simulink library "tqd"  (R2021b)
settings: Solver=VariableStepAuto  StartTime=0.0  StopTime=10.0  RelTol=1e-3
undefined symbols (not defined in the file or in its folder): ATQD_APSDecReq_X_kph, ATQD_APSDecReq_Y_mps2, ATQD_APSDecReqCMD_X_kph, ATQD_APSDecReqTs_X_pct, ATQD_APSDecTimeGain_X_Deg, ATQD_APSDecTimeGain_Y_s, ATQD_APSReqLowSpd_X_Deg, ATQD_AutoHoldReleaseBPS_X_Deg, ATQD_AWDLoadTrqnsGain_X_kg, ATQD_AWDLoadTrqnsGain_Y_pct, ATQD_BOSEnBPSPosn_X_kph, ATQD_BOSMap_X_rpm, ATQD_BOSMap_Y_pct, ATQD_CreepBaseTqD_X_kph, ATQD_CreepBaseTqD_Y_Deg, ATQD_CreepBaseTqR_X_kph, ATQD_CreepBaseTqR_Y_Deg, ATQD_CreepBPSDisPosn_X_Deg, ATQD_CreepBPSDisPosnR_X_Deg, ATQD_CreepBPSEnPosn_X_Deg, ATQD_CreepBPSEnPosnR_X_Deg, ATQD_CreepDeltaTq_X_kph, ATQD_CreepIterm_X_kph, ATQD_CreepIterm_Y_kph, ATQD_CreepItermMaxLimit_X_pct, ATQD_CreepPreloadTime_X_kph, ATQD_CreepPreloadTq_X_kph, ATQD_CreepPreloadTq_Y_s, ATQD_CreepProtTq_X_Deg, ATQD_CreepPterm_X_kph, ATQD_ECOTqMapD_X_rpm, ATQD_ECOTqMapD_Y_pct, ATQD_EOPDTqMapDCon_X_rpm, ATQD_EOPDTqMapDCon_Y_Deg, ATQD_EstInitVehWeight_X_c, ATQD_LHMRollGenMapD_X_rpm, ATQD_LHMRollGenMapD_Y_rpm, ATQD_LHMTqMapD_X_rpm, ATQD_LHMTqMapD_Y_pct, ATQD_NL1TqMapD_X_rpm, ATQD_NL1TqMapD_Y_pct, ATQD_NOPDTqMapDCon_X_rpm, ATQD_NOPDTqMapDCon_Y_Deg, ATQD_NRMRrEDUSpRat_X_rpm, ATQD_NRMRrEDUSpRat_Y_Nm, ATQD_OPDHoldDownRelDelay_X_Deg, ATQD_OPDHoldEnSpd_X_Deg, ATQD_OPDHoldRelDetTime_X_Deg, ATQD_OPDHoldReleaseTq_X_Deg, ATQD_OrigPedTqLowLim_X_Deg, ATQD_OrigPedTqLowLim_Y_pct, ATQD_PedalMapClimbUpLim_X_rpm, ATQD_PedalMapClimbUpLim_Y_Deg, ATQD_PreLoadTq_X_s, ATQD_RollGenMapEL1_X_rpm, ATQD_RollGenMapEL1_Y_rpm, ATQD_SL1TqMapD_X_rpm, ATQD_SL1TqMapD_Y_pct, ATQD_SlideRegenTqGain_X_Gps, ATQD_SlideRegenTqGain_Y_pct ... (+378)
libraries: hcu_lib x59, simulink x49
(part 3 of 12)

== system tqd/TQD/TorqueDemand/ShiftModule ==
  task_time_s : Inport
  VINP_ShifterHandleCmd_enum : Inport  Port=2
  VINP_VehSpeed_kph : Inport  Port=3
  VTQD_BrkSwSta_flg : Inport  Port=4
  VPMM_PowerSta_enum : Inport  Port=5
  VINP_PBWMotorPos_enum : Inport  Port=6
  VTQD_TMRotateDirction_enum : Inport  Port=7
  VTQD_EPBCarWashMode_flg : Inport  Port=8
  VINP_DrDoorSW_flg : Inport  Port=9
  VVMC_APSShiftPosnReq_enum : Inport  Port=10
  VVMC_APSActive_flg : Inport  Port=11
  VINP_DriverSeatBeltCmd_flg : Inport  Port=12
  VINP_SeatSW_flg : Inport  Port=13
  VINP_ChrgPlugSta_enum : Inport  Port=14
  VINP_SCPSystemMode_enum : Inport  Port=15
  VTQD_AfterAvailableTqDemFr_Nm : Inport  Port=16
  VTQD_AfterAvailableTqDemRr_Nm : Inport  Port=17
  VTQR_NoABSFEDUWhlTqReq_Nm : Inport  Port=18
  VTQR_NoABSREDUWhlTqReq_Nm : Inport  Port=19
  VINP_DOASta_flg : Inport  Port=20
  VTQD_IVIPwrLock_flg : Inport  Port=21
  VTQD_OPDHoldAllowPark_flg : Inport  Port=22
  Constant : Constant  Value=KTQD_VehSpd2P_kph
  Constant1 : Constant  Value=KTQD_PBWTimeout_s
  Constant2 : Constant  Value=KTQD_VehSpdRev_kph
  Constant3 : Constant  Value=KTQD_ShiftInitialTime_s
  Constant4 : Constant  Value=KTQD_RelockWaitTime_s
  Constant5 : Constant  Value=KTQD_ReunlockWaitTime_s
  Constant6 : Constant  Value=ENUM_GEARACTUALPOSN_P
  Constant7 : Constant  Value=ENUM_GEARACTUALPOSN_P
  Data Type Conversion1 : DataTypeConversion
  Data Type Conversion2 : DataTypeConversion
  Data Type Conversion3 : DataTypeConversion  OutDataTypeStr=uint8
  Data Type Conversion4 : DataTypeConversion  OutDataTypeStr=boolean
  Determine_Actual_Gear_Position : Stateflow chart  TreatAsAtomicUnit=on
  Equal : RelationalOperator  Operator===  OutDataTypeStr=boolean  RndMeth=Simplest
  Equal1 : RelationalOperator  Operator=~=  OutDataTypeStr=boolean  RndMeth=Simplest
  GearShiftPosn : Subsystem  Description=GearPosition
  P_Button_State_Judge : Subsystem
  SR_Latch : hcu_lib/Basic_Blocks/SR_Latch
  SR_Latch1 : Subsystem  mask(SR_Latch){}
      mask help: SR latch function.
  Terminator : Terminator
  VTQD_GearActualPosn_enum : Outport
  VTQD_ParkRequest_flg : Outport  Port=2
  VTQD_PBWLockTO_flg : Outport  Port=3
  VTQD_PBWUnlockTO_flg : Outport  Port=4
  VTQD_PButtonSta_enum : Outport  Port=5
  VTQD_DriveProtRemove_flg : Outport  Port=6
  VTQD_DriveProtEn_flg : Outport  Port=7
  wires:
  VPMM_PowerSta_enum/1 -> [VPMM_PowerSta_enum]
  task_time_s/1 -> [task_time_s]
  VINP_VehSpeed_kph/1 -> [VINP_VehSpeed_kph]
  VTQD_BrkSwSta_flg/1 -> [VTQD_BrkSwSta_flg]
  VTQD_TMRotateDirction_enum/1 -> [VTQD_TMRotateDirction_enum]
  VINP_PBWMotorPos_enum/1 -> [VINP_PBWMotorPos_enum]
  P_Button_State_Judge/1(VTQD_PButtonSta_enum) -> VTQD_PButtonSta_enum/1
  VINP_ShifterHandleCmd_enum/1 -> [VINP_ShifterHandleCmd_enum]
  [VINP_ShifterHandleCmd_enum] -> P_Button_State_Judge/1(VINP_ShifterHandleCmd_enum)
  VINP_SCPSystemMode_enum/1 -> Terminator/1
  VINP_ChrgPlugSta_enum/1 -> [VINP_ChrgPlugSta_enum]
  VINP_SeatSW_flg/1 -> [VINP_SeatSW_flg]
  VINP_DriverSeatBeltCmd_flg/1 -> [VINP_DriverSeatBeltCmd_flg]
  VVMC_APSActive_flg/1 -> [VVMC_APSActive_flg]
  VVMC_APSShiftPosnReq_enum/1 -> [VVMC_APSShiftPosnReq_enum]
  VINP_DrDoorSW_flg/1 -> [VINP_DrDoorSW_flg]
  VTQD_EPBCarWashMode_flg/1 -> [VTQD_EPBCarWashMode_flg]
  [VTQD_EPBCarWashMode_flg] -> GearShiftPosn/8(VTQD_EPBCarWashMode_flg)
  [VINP_VehSpeed_kph] -> GearShiftPosn/9(VINP_VehSpeed_kph)
  [VINP_ChrgPlugSta_enum] -> GearShiftPosn/10(VINP_ChrgPlugSta_enum)
  GearShiftPosn/3(VTQD_PwrStaAllowDR_flg) -> [VTQD_PwrStaAllowDR_flg]
  [VVMC_APSShiftPosnReq_enum] -> GearShiftPosn/4(VVMC_APSShiftPosnReq_enum)
  [VINP_DrDoorSW_flg] -> GearShiftPosn/3(VINP_DrDoorSW_flg)
  [VINP_ShifterHandleCmd_enum] -> GearShiftPosn/1(VINP_ShifterHandleCmd_enum)
  [VVMC_APSActive_flg] -> GearShiftPosn/5(VVMC_APSActive_flg)
  [VINP_DriverSeatBeltCmd_flg] -> GearShiftPosn/6(VINP_DriverSeatBeltCmd_flg)
  GearShiftPosn/1(VTQD_GearShiftCMD_enum) -> [VTQD_GearShiftCMD_enum]
  [VINP_SeatSW_flg] -> GearShiftPosn/7(VINP_SeatSW_flg)
  [VPMM_PowerSta_enum] -> GearShiftPosn/2(VPMM_PowerSta_enum)
  GearShiftPosn/2(VTQD_PwrStaAllowPN_flg) -> [VTQD_PwrStaAllowPN_flg]
  Data Type Conversion4/1 -> VTQD_ParkRequest_flg/1  "VTQD_ParkRequest_flg"
  Constant6/1 -> Equal/2
  Data Type Conversion1/1 -> SR_Latch/1
  [VTQD_GearActualPosn_enum] -> Equal1/1
  [VTQD_GearActualPosn_enum] -> Equal/1
  Data Type Conversion2/1 -> SR_Latch1/1(set)
  Determine_Actual_Gear_Position/4(VTQD_ParkRequest_flg) -> Data Type Conversion4/1
  Constant7/1 -> Equal1/2
  Data Type Conversion3/1 -> [VTQD_GearActualPosn_enum], VTQD_GearActualPosn_enum/1  "VTQD_GearActualPosn_enum"
  Determine_Actual_Gear_Position/3(VTQD_PBWUnlockTO_flg) -> Data Type Conversion2/1
  SR_Latch1/1(latched) -> VTQD_PBWUnlockTO_flg/1  "VTQD_PBWUnlockTO_flg"
  Equal1/1 -> SR_Latch1/2(reset)
  Equal/1 -> SR_Latch/2
  Determine_Actual_Gear_Position/2(VTQD_PBWLockTO_flg) -> Data Type Conversion1/1
  Determine_Actual_Gear_Position/1(VTQD_GearActualPosn_enum) -> Data Type Conversion3/1
  SR_Latch/1 -> VTQD_PBWLockTO_flg/1  "VTQD_PBWLockTO_flg"
  [VTQD_GearActualPosn_enum] -> GearShiftPosn/11(VTQD_GearActualPosn_enum)
  [VTQD_AfterAvailableTqDemFr_Nm] -> GearShiftPosn/12(VTQD_AfterAvailableTqDemFr_Nm)
  [VTQR_NoABSREDUWhlTqReq_Nm] -> GearShiftPosn/15(VTQR_NoABSREDUWhlTqReq_Nm)
  [VTQR_NoABSFEDUWhlTqReq_Nm] -> GearShiftPosn/14(VTQR_NoABSFEDUWhlTqReq_Nm)
  [VTQD_AfterAvailableTqDemRr_Nm] -> GearShiftPosn/13(VTQD_AfterAvailableTqDemRr_Nm)
  [task_time_s] -> GearShiftPosn/16(task_time_s)
  VTQD_AfterAvailableTqDemFr_Nm/1 -> [VTQD_AfterAvailableTqDemFr_Nm]
  VTQD_AfterAvailableTqDemRr_Nm/1 -> [VTQD_AfterAvailableTqDemRr_Nm]
  VTQR_NoABSFEDUWhlTqReq_Nm/1 -> [VTQR_NoABSFEDUWhlTqReq_Nm]
  VTQR_NoABSREDUWhlTqReq_Nm/1 -> [VTQR_NoABSREDUWhlTqReq_Nm]
  VINP_DOASta_flg/1 -> [VINP_DOASta_flg]
  [VINP_DOASta_flg] -> GearShiftPosn/17(VINP_DOASta_flg)
  GearShiftPosn/4(VTQD_DriveProtRemove_flg) -> VTQD_DriveProtRemove_flg/1
  GearShiftPosn/5(VTQD_DriveProtEn_flg) -> VTQD_DriveProtEn_flg/1
  VTQD_IVIPwrLock_flg/1 -> [VTQD_IVIPwrLock_flg]
  [VTQD_IVIPwrLock_flg] -> GearShiftPosn/18(VTQD_IVIPwrLock_flg)
  [VTQD_BrkSwSta_flg] -> GearShiftPosn/19(VTQD_BrkSwSta_flg)
  GearShiftPosn/6(VTQD_ForceP_flg) -> [VTQD_ForceP_flg]
  Constant/1 -> Determine_Actual_Gear_Position/9(KTQD_VehSpd2P_kph)
  [VTQD_ForceP_flg] -> Determine_Actual_Gear_Position/17(VTQD_ForceP_flg)
  [VINP_VehSpeed_kph] -> Determine_Actual_Gear_Position/4(VINP_VehSpd_kph)
  [VINP_PBWMotorPos_enum] -> Determine_Actual_Gear_Position/5(VINP_PBWMotorPos_enum)
  Constant5/1 -> Determine_Actual_Gear_Position/14(KTQD_ReunlockWaitTime_s)
  [VTQD_PwrStaAllowDR_flg] -> Determine_Actual_Gear_Position/6(VTQD_PwrStaAllowDR_flg)
  [VTQD_BrkSwSta_flg] -> Determine_Actual_Gear_Position/2(VTQD_BrkSwSta_flg)
  [task_time_s] -> Determine_Actual_Gear_Position/1(task_time_s)
  Constant1/1 -> Determine_Actual_Gear_Position/12(KTQD_PBWTimeout_s)
  [VTQD_PwrStaAllowPN_flg] -> Determine_Actual_Gear_Position/7(VTQD_PwrStaAllowPN_flg)
  Constant4/1 -> Determine_Actual_Gear_Position/13(KTQD_RelockWaitTime_s)
  [VTQD_GearShiftCMD_enum] -> Determine_Actual_Gear_Position/3(VTQD_GearShiftCMD_enum)
  [VVMC_APSActive_flg] -> Determine_Actual_Gear_Position/16(VVMC_APSActive_flg)
  [VTQD_TMRotateDirction_enum] -> Determine_Actual_Gear_Position/8(VTQD_TMRotateDirction_enum)
  Constant3/1 -> Determine_Actual_Gear_Position/11(KTQD_ShiftInitialTime_s)
  Constant2/1 -> Determine_Actual_Gear_Position/10(KTQD_VehSpdRev_kph)
  [VTQD_EPBCarWashMode_flg] -> Determine_Actual_Gear_Position/15(VINP_EPBCarWashMode_flg)
  [VTQD_OPDHoldAllowPark_flg] -> GearShiftPosn/20(VTQD_OPDHoldAllowPark_flg)
  VTQD_OPDHoldAllowPark_flg/1 -> [VTQD_OPDHoldAllowPark_flg]

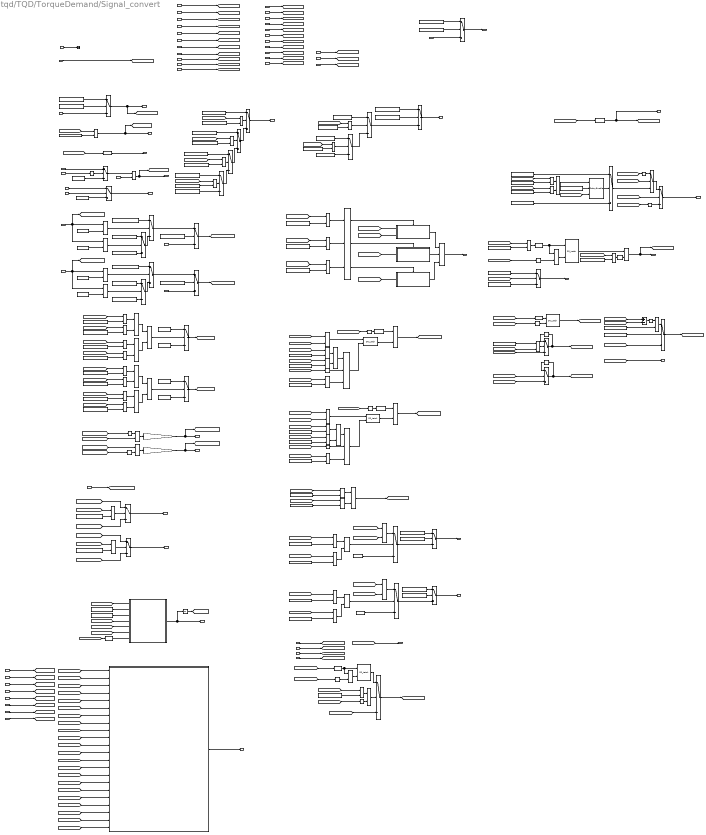
== system tqd/TQD/TorqueDemand/Signal_convert ==
  note: LowIdle Acc Pedal
  note: Equivalent Acceleration Pedal Switch signal
  note: Creep function switch2
  note: %VINP_IVIPWModeReq_enum
      | ENUM_IVIPWMODEREQ_NRM = uint8( 0 );
      | ENUM_IVIPWMODEREQ_SPORT = uint8( 1 );
      | ENUM_IVIPWMODEREQ_ECO = uint8( 2 ); ENUM_IVIPWMODEREQ_NOREQUEST = uint8( 3 );
  note: % VTQD_EVDriveMode_enum
      | ENUM_DRIVEMODE_NRM = uint8( 0 );
      | ENUM_DRIVEMODE_ECO = uint8( 1 );
      | ENUM_DRIVEMODE_SPORT = uint8( 2 );
      | ENUM_DRIVEMODE_LAUNCH = uint8( 3 );
  note: Driving mode determination
  note: MCU Damping Disable Judgement
  note: Actual gear position signal defination converter for CAN bus
  note: Fr and Rr Wheel Rotate Diraction Detect
  note: Fr and Rr Wheel Rotate Diraction Detect
  note: Brake pedal signal handle
  note: Rolling Regen Cancel Request Handle
  note: APS Position Handle
  note: Target Shaft Speed and Direction Judgement
  note: MCU Ready for External judgement
  note: Regen Drag Control (RDC) signal
  note: VINP_EPBCarWashMode_flg
  note: Exhibition Status
  note: Regen Mode Latch
  VTQD_GearActualPosn_enum : Inport
  VDHP_LowIdleAccPedal_flg : Inport  Port=2
  VDHP_ActAPSPosn_pct : Inport  Port=3
  VINP_BrkSwSta_flg : Inport  Port=4
  VINP_BrakeSWGPIO_flg : Inport  Port=5
  VINP_BrkSwV_flg : Inport  Port=6
  VINP_BrkPedalPos_pct : Inport  Port=7
  VINP_BrkPedalPosSta_flg : Inport  Port=8
  VINP_FrTMSpd_rpm : Inport  Port=9
  VINP_RrTMSpd_rpm : Inport  Port=10
  VPMM_DrivetrainSelect_enum : Inport  Port=11
  VINP_FrEDURotateDirction_enum : Inport  Port=12
  VINP_RrEDURotateDirction_enum : Inport  Port=13
  VDDM_LimpHomeAct_flg : Inport  Port=14
  VINP_CreepSW_flg : Inport  Port=15
  VINP_VehSpeed_kph : Inport  Port=16
  VINP_IVIPWModeReq_enum : Inport  Port=17
  VINP_MCUWarnF_enum : Inport  Port=18
  VINP_MCUWarnR_enum : Inport  Port=19
  task_time_s : Inport  Port=20
  VINP_FrEDURealTMTq_Nm : Inport  Port=21
  VINP_RrEDURealTMTq_Nm : Inport  Port=22
  VINP_IVICreepSWReq_flg : Inport  Port=23
  VPMM_SysPowerMode_enum : Inport  Port=24
  VTQD_OPDOn2Off_flg : Inport  Port=25
  VINP_RegenMode_enum : Inport  Port=26
  VINP_FrntAxlTrqReqBrk_Nm : Inport  Port=27
  VINP_RearAxlTrqReqBrk_Nm : Inport  Port=28
  VINP_FrRBCActive_flg : Inport  Port=29
  VINP_RrRBCActive_flg : Inport  Port=30
  VVMC_ADASActive_flg : Inport  Port=31
  VINP_ACCRequiredAccel_mps2 : Inport  Port=32
  VVMC_ACCPedalOvrd_flg : Inport  Port=33
  VTQD_AfterAvailableTqDemFr_Nm : Inport  Port=34
  VTQD_AfterAvailableTqDemRr_Nm : Inport  Port=35
  VVMC_ADASWhlTqReq_Nm : Inport  Port=36
  VTQR_NoABSREDUWhlTqReq_Nm : Inport  Port=37
  VTQR_NoABSFEDUWhlTqReq_Nm : Inport  Port=38
  VVMC_LongAcc_Gps : Inport  Port=39
  VINP_DriverSeatBeltCmd_flg : Inport  Port=40
  VINP_PsngrSeatBeltCmd_flg : Inport  Port=41
  VINP_RDriverSeatBeltCmd_flg : Inport  Port=42
  VINP_RCenterSeatBeltCmd_flg : Inport  Port=43
  VINP_RPsngrSeatBeltCmd_flg : Inport  Port=44
  VINP_RollModeSWCmd_enum : Inport  Port=45
  VINP_SCPSystemMode_enum : Inport  Port=46
  VINP_EPBCarWashMode_flg : Inport  Port=47
  VINP_DOASta_flg : Inport  Port=48
  VVMC_EstSlope_Deg : Inport  Port=49
  VINP_IVIPwrLockSW_enum : Inport  Port=50
  VVMC_RWDRDCActive_enum : Inport  Port=51
  AND{,3..5} (4 alike) : Logic  AllPortsSameDT=off  OutDataTypeStr=boolean
  AND1 : Logic  Operator=OR  AllPortsSameDT=off  OutDataTypeStr=boolean
  AND2 : Logic  Operator=OR  AllPortsSameDT=off  OutDataTypeStr=boolean
  AND9 : Logic  Operator=OR  AllPortsSameDT=off  OutDataTypeStr=boolean
  AWDMCUReadyExt_flg : Subsystem  TreatAsAtomicUnit=on
  Abs : Abs
  Abs1 : Abs
  Abs2 : Abs
  Add : Sum  Inputs=+-
  Chart : Stateflow chart  TreatAsAtomicUnit=on
  Constant{,45,61..62} (4 alike) : Constant  Value=FALSE
  Constant1 : Constant  Value=KTQD_RgnModeChgResetSW_flg
  Constant10 : Constant  Value=ENUM_GEARACTUALPOSN_D
  Constant{11,14,30,35} (4 alike) : Constant  Value=ENUM_TMROTATEDIRECTACT_REVERSE  OutDataTypeStr=Inherit: Inherit via back propagation
  Constant12 : Constant  Value=ENUM_TMROTATEDIRECTACT_STOP  OutDataTypeStr=Inherit: Inherit via back propagation
  Constant13 : Constant  Value=ZERO_FLOAT
  Constant15 : Constant  Value=ENUM_TMROTATEDIRECTACT_STOP  OutDataTypeStr=Inherit: Inherit via back propagation
  Constant16 : Constant  Value=KTQD_DriveModeReq_enum_ovrdflg  OutDataTypeStr=Inherit: Inherit via back propagation
  Constant17 : Constant  Value=KTQD_DriveModeReq_enum_ovrdval  OutDataTypeStr=Inherit: Inherit via back propagation
  Constant{5,18,20,23} (4 alike) : Constant  Value=ZERO_FLOAT  OutDataTypeStr=Inherit: Inherit via back propagation
  Constant19 : Constant  Value=KTQD_AbsoluteMotorSpdDir_flg  OutDataTypeStr=Inherit: Inherit via back propagation
  Constant2 : Constant  Value=ENUM_RDCACTSTA_NOREQUEST
  Constant{6,21,48,76} (4 alike) : Constant  Value=ENUM_DRIVETRAIN_FWD
  Constant22 : Constant  Value=KTQD_AbsoluteMotorSpdDir_flg  OutDataTypeStr=Inherit: Inherit via back propagation
  Constant24 : Constant  Value=KTQD_MCUDmEnFrBrkTq_Nm
  Constant25 : Constant  Value=KTQD_MCUDmEnAccCMD_mps2
  Constant26 : Constant  Value=TRUE
  Constant27 : Constant  Value=KTQD_MCUDmEnRrBrkTq_Nm
  Constant{7,28,32,37} (4 alike) : Constant  Value=ENUM_TMROTATEDIRECTACT_FORWARD  OutDataTypeStr=Inherit: Inherit via back propagation
  Constant29 : Constant  Value=ENUM_GEARACTUALPOSN_D
  Constant3 : Constant  Value=KTQD_LimpHomeAct_flg_ovrdflg  OutDataTypeStr=Inherit: Inherit via back propagation
  Constant31 : Constant  Value=ENUM_GEARACTUALPOSN_R
  Constant33 : Constant  Value=ONE_FLOAT
  Constant34 : Constant  Value=MINUSONE_FLOAT
  Constant36 : Constant  Value=ENUM_GEARACTUALPOSN_R
  Constant38 : Constant  Value=ONE_FLOAT
  Constant39 : Constant  Value=MINUSONE_FLOAT
  Constant4 : Constant  Value=KTQD_LimpHomeAct_flg_ovrdval  OutDataTypeStr=Inherit: Inherit via back propagation
  Constant40 : Constant  Value=KTQD_ActvDmpDisabAPSPosn_pct  OutDataTypeStr=Inherit: Inherit via back propagation
  Constant41 : Constant  Value=KTQD_ActvDmpDisabVehSpd_kph  OutDataTypeStr=Inherit: Inherit via back propagation
  Constant42 : Constant  Value=KTQD_LowIdle_flg_ovrdflg  OutDataTypeStr=Inherit: Inherit via back propagation
  Constant43 : Constant  Value=KTQD_LowIdle_flg_ovrdval  OutDataTypeStr=Inherit: Inherit via back propagation
  Constant44 : Constant  Value=KTQD_MCUDmEnAccCMD_mps2
  Constant46 : Constant  Value=ENUM_DRIVEMODE_NRM
  Constant47 : Constant  Value=ENUM_IVIPWMODEREQ_SPORT
  Constant49 : Constant  Value=ENUM_DRIVETRAIN_AWD
  Constant50 : Constant  Value=ENUM_GEARPOSNTOCAN_N  OutDataTypeStr=Inherit: Inherit via back propagation
  Constant51 : Constant  Value=ENUM_GEARPOSNTOCAN_D  OutDataTypeStr=Inherit: Inherit via back propagation
  Constant52 : Constant  Value=ENUM_GEARPOSNTOCAN_FAIL  OutDataTypeStr=Inherit: Inherit via back propagation
  Constant53 : Constant  Value=ENUM_GEARACTUALPOSN_D
  Constant54 : Constant  Value=ENUM_GEARACTUALPOSN_N
  Constant55 : Constant  Value=ENUM_GEARPOSNTOCAN_R  OutDataTypeStr=Inherit: Inherit via back propagation
  Constant56 : Constant  Value=ENUM_GEARACTUALPOSN_R
  Constant57 : Constant  Value=ENUM_GEARPOSNTOCAN_P  OutDataTypeStr=Inherit: Inherit via back propagation
  Constant58 : Constant  Value=ENUM_GEARACTUALPOSN_P
  Constant59 : Constant  Value=ENUM_DRIVETRAIN_RWD
  Constant60 : Constant  Value=ENUM_DRIVETRAIN_AWD
  Constant63 : Constant  Value=KTQD_RrDmpDisabReq_flg_ovrdval  OutDataTypeStr=Inherit: Inherit via back propagation
  Constant64 : Constant  Value=KTQD_FrDmpDisabReq_flg_ovrdval  OutDataTypeStr=Inherit: Inherit via back propagation
  Constant65 : Constant  Value=KTQD_MCUDmEnRrBrkTq_Nm
  Constant66 : Constant  Value=ENUM_SYSMODE_MANUFACTURE
  Constant67 : Constant  Value=KTQD_FrDmpDisabReq_flg_ovrdflg  OutDataTypeStr=Inherit: Inherit via back propagation
  Constant68 : Constant  Value=KTQD_RrDmpDisabReq_flg_ovrdflg  OutDataTypeStr=Inherit: Inherit via back propagation
  Constant69 : Constant  Value=ENUM_DRIVEMODE_ECO
  Constant70 : Constant  Value=ENUM_IVIPWMODEREQ_ECO
  Constant71 : Constant  Value=ENUM_DRIVEMODE_SPORT
  Constant72 : Constant  Value=ENUM_DRIVETRAIN_RWD
  Constant73 : Constant  Value=KTQD_RgnModeChgResetAPSDev_pct
  Constant74 : Constant  Value=KTQD_RgnModeChgSW_flg
  Constant75 : Constant  Value=ENUM_DRIVETRAIN_AWD
  Constant77 : Constant  Value=ENUM_GEARACTUALPOSN_P
  Constant79 : Constant  Value=KTQD_CreepSW_flg_ovrdflg
  Constant8 : Constant  Value=KTQD_ADASLowIdleWhlTq_Nm
  Constant80 : Constant  Value=KTQD_CreepSW_flg_ovrdval
  Constant85 : Constant  Value=KTQD_ACCReqCMdBond_mps2
  Constant9 : Constant  Value=KTQD_MCUDmEnFrBrkTq_Nm
  Constant93 : Constant  Value=KTQD_EquivAccPedalDelay_s
  Constant96 : Constant  Value=ENUM_IVIPWRLOCKSW_PRESS
  Constant97 : Constant  Value=ENUM_PWRLOCKSta_LOCKED
  Constant98 : Constant  Value=ENUM_PWRLOCKSta_UNLOCKED
  Data Type Conversion : DataTypeConversion  OutDataTypeStr=boolean
  Data Type Conversion1 : DataTypeConversion  OutDataTypeStr=boolean
  Data Type Conversion2 : DataTypeConversion
  Data Type Conversion3 : DataTypeConversion
  Delay{,1..4,8} (6 alike) : Delay  DelayLength=1
  DelayEnable4 : hcu_lib/Basic_Blocks/DelayEnable
  Detect Change : simulink/Logic and Bit Operations/Detect Change  vinit=0  OutDataTypeStr=boolean
  Detect Decrease : simulink/Logic and Bit Operations/Detect Decrease  vinit=0.0  OutDataTypeStr=boolean
  Detect Decrease4 : simulink/Logic and Bit Operations/Detect Decrease  vinit=0.0  OutDataTypeStr=boolean
  Detect Decrease5 : simulink/Logic and Bit Operations/Detect Decrease  vinit=0.0  OutDataTypeStr=boolean
  Equal{,1..19,21..23,30,32,34} (26 alike) : RelationalOperator  Operator===  OutDataTypeStr=boolean  RndMeth=Simplest
  Equal20 : RelationalOperator  Operator=~=  OutDataTypeStr=boolean  RndMeth=Simplest
  Equal{24..25,27..28} (4 alike) : RelationalOperator  OutDataTypeStr=boolean  RndMeth=Simplest
  Equal26 : RelationalOperator  Operator=>  OutDataTypeStr=boolean  RndMeth=Simplest
  Equal29 : RelationalOperator  Operator=>  OutDataTypeStr=boolean  RndMeth=Simplest
  FWDMCUReadyExt_flg : Subsystem  TreatAsAtomicUnit=on
  Gain : Gain  Gain=1/KTQD_FrTMTotalGearRatio_gain
  Gain2 : Gain  Gain=1/KTQD_RrTMTotalGearRatio_gain
  GreaterThan : RelationalOperator  Operator=>  OutDataTypeStr=boolean  RndMeth=Simplest
  GreaterThan1 : RelationalOperator  Operator=<  OutDataTypeStr=boolean  RndMeth=Simplest
  GreaterThan2 : RelationalOperator  Operator=>  OutDataTypeStr=boolean  RndMeth=Simplest
  GreaterThan3 : RelationalOperator  Operator=<  OutDataTypeStr=boolean  RndMeth=Simplest
  If : If  NumInputs=3  IfExpression=u1 ~= 0  ElseIfExpressions=u2 ~= 0
  Less Than : RelationalOperator  Operator=<=  OutDataTypeStr=boolean  RndMeth=Simplest
  Less Than1 : RelationalOperator  Operator=<=  OutDataTypeStr=boolean  RndMeth=Simplest
  LiuzgSwitch{2..13,15..17,19..22} (19 alike) : Switch  Criteria=u2 ~= 0
      settings: AttributesFormatString=<%<Criteria>>
  Logical Operator{,2..3,5,7,10,12..13,15,17..18} (11 alike) : Logic  AllPortsSameDT=off  OutDataTypeStr=boolean
  Logical Operator{1,4,8,19} (4 alike) : Logic  Operator=OR  AllPortsSameDT=off  OutDataTypeStr=boolean
  Logical Operator11 : Logic  Operator=OR  Inputs=3  AllPortsSameDT=off  OutDataTypeStr=boolean
  Logical Operator14 : Logic  Operator=OR  Inputs=3  AllPortsSameDT=off  OutDataTypeStr=boolean
  Logical Operator{6,9,16,21..22} (5 alike) : Logic  Operator=NOT  AllPortsSameDT=off  OutDataTypeStr=boolean
  Merge : Merge  Inputs=3
  NOT : Logic  Operator=NOT  AllPortsSameDT=off  OutDataTypeStr=boolean
  OR : Logic  Operator=OR  AllPortsSameDT=off  OutDataTypeStr=boolean
  OR1 : Logic  Operator=OR  AllPortsSameDT=off  OutDataTypeStr=boolean
  Product2 : Product
  Product3 : Product
  RWDMCUReadyExt_flg : Subsystem  TreatAsAtomicUnit=on
  Relational Operator : RelationalOperator  OutDataTypeStr=boolean  RndMeth=Simplest
  Relational Operator1 : RelationalOperator  Operator=>  OutDataTypeStr=boolean  RndMeth=Simplest
  Relational Operator5 : RelationalOperator  OutDataTypeStr=boolean  RndMeth=Simplest
  Relay : Relay  OnSwitchValue=KTQD_FrMCUDmDisSpd_kph  OffSwitchValue=KTQD_FrMCUDmEnSpd_kph
      settings: AttributesFormatString=|
      | ON : %<OffSwitchValue>
      | OFF : %<OnSwitchValue>
  Relay1 : Relay  OnSwitchValue=KTQD_RrMCUDmDisSpd_kph  OffSwitchValue=KTQD_RrMCUDmEnSpd_kph
      settings: AttributesFormatString=|
      | ON : %<OffSwitchValue>
      | OFF : %<OnSwitchValue>
  SR_Latch{,1..3,6} (5 alike) : hcu_lib/Basic_Blocks/SR_Latch
  Switch : Switch  Criteria=u2 ~= 0
  Switch1 : Switch  Criteria=u2 ~= 0
  Switch{8,10..12,14} (5 alike) : Switch  Criteria=u2 > Threshold
  Switch{2..6,9} (6 alike) : Switch  Criteria=u2 ~= 0  Threshold=0.5
      settings: AttributesFormatString=%<Criteria>
  Switch7 : Switch  Criteria=u2 ~= 0
  Terminator : Terminator
  Unit Delay1 : UnitDelay  SampleTime=-1  HasFrameUpgradeWarning=on
  VehWeightEst : Subsystem
  VTQD_LowIdleAccPedal_flg : Outport
  VTQD_RollRegenDisable_flg : Outport  Port=2
  VTQD_ActAPSPosn_pct : Outport  Port=3
  VTQD_BrkSwSta_flg : Outport  Port=4
  VTQD_ActBPSPosn_pct : Outport  Port=5
  VTQD_FrShaftSpd_rpm : Outport  Port=6
  VTQD_RrShaftSpd_rpm : Outport  Port=7
  VTQD_TqTargetShaftSpd_rpm : Outport  Port=8
  VTQD_TMRotateDirction_enum : Outport  Port=9
  VTQD_LimpHomeAct_flg : Outport  Port=10
  VTQD_EVDriveMode_enum : Outport  Port=11
  VTQD_CreepON_flg : Outport  Port=12
  VTQD_ShiftGearPosn_enum : Outport  Port=13
  VTQD_FrActvDmpDisabReq_flg : Outport  Port=14
  VTQD_RrActvDmpDisabReq_flg : Outport  Port=15
  VTQD_MCUReady4Ext_flg : Outport  Port=16
  VTQD_EstVehWeightResult_kg : Outport  Port=17
  VTQD_RDCActive_enum : Outport  Port=18
  VTQD_EquivAccPedalSWSta_flg : Outport  Port=19
  VTQD_EPBCarWashMode_flg : Outport  Port=20
  VTQD_IVIPwrLock_flg : Outport  Port=21
  VTQD_IVIPwrLockSta_enum : Outport  Port=22
  VTQD_RegenMode_enum : Outport  Port=23
  wires:
  Constant17/1 -> Switch3/1
  Constant16/1 -> Switch3/2
  Switch3/1 -> VTQD_EVDriveMode_enum/1  "VTQD_EVDriveMode_enum"
  Constant4/1 -> Switch2/1
  Constant3/1 -> Switch2/2
  VDDM_LimpHomeAct_flg/1 -> Switch2/3
  Switch2/1 -> VTQD_LimpHomeAct_flg/1  "VTQD_LimpHomeAct_flg"
  Equal8/1 -> LiuzgSwitch7/2
  [VPMM_DrivetrainSelect_enum] -> Equal8/1
  Constant21/1 -> Equal8/2
  [VTQD_FrShaftSpd_rpm] -> LiuzgSwitch7/1
  [VTQD_RrShaftSpd_rpm] -> LiuzgSwitch7/3
  LiuzgSwitch7/1 -> VTQD_TqTargetShaftSpd_rpm/1  "VTQD_TqTargetShaftSpd_rpm"
  Constant5/1 -> GreaterThan/2
  Constant7/1 -> LiuzgSwitch2/1
  GreaterThan/1 -> LiuzgSwitch2/2
  GreaterThan1/1 -> LiuzgSwitch3/2
  Constant18/1 -> GreaterThan1/2
  VINP_FrTMSpd_rpm/1 -> GreaterThan1/1, GreaterThan/1, [VINP_FrTMSpd_rpm]
  LiuzgSwitch3/1 -> LiuzgSwitch2/3
  Constant11/1 -> LiuzgSwitch3/1
  Constant12/1 -> LiuzgSwitch3/3
  Constant19/1 -> LiuzgSwitch4/2
  LiuzgSwitch2/1 -> LiuzgSwitch4/1
  LiuzgSwitch4/1 -> [VTQD_FrTMRotateDirction_enum]
  VINP_BrkSwV_flg/1 -> Logical Operator6/1
  VINP_BrkSwSta_flg/1 -> LiuzgSwitch5/1
  Constant/1 -> LiuzgSwitch5/3
  VINP_BrkPedalPos_pct/1 -> LiuzgSwitch6/1
  VINP_BrkPedalPosSta_flg/1 -> LiuzgSwitch6/2
  LiuzgSwitch6/1 -> VTQD_ActBPSPosn_pct/1  "VTQD_ActBPSPosn_pct"
  Constant13/1 -> LiuzgSwitch6/3
  VINP_FrEDURotateDirction_enum/1 -> LiuzgSwitch4/3
  VINP_RrEDURotateDirction_enum/1 -> LiuzgSwitch10/3
  LiuzgSwitch10/1 -> [VTQD_RrTMRotateDirction_enum]
  LiuzgSwitch8/1 -> LiuzgSwitch10/1
  Constant22/1 -> LiuzgSwitch10/2
  Constant15/1 -> LiuzgSwitch9/3
  Constant14/1 -> LiuzgSwitch9/1
  LiuzgSwitch9/1 -> LiuzgSwitch8/3
  VINP_RrTMSpd_rpm/1 -> [VINP_RrTMSpd_rpm], GreaterThan2/1, GreaterThan3/1
  Constant20/1 -> GreaterThan3/2
  GreaterThan3/1 -> LiuzgSwitch9/2
  GreaterThan2/1 -> LiuzgSwitch8/2
  Constant28/1 -> LiuzgSwitch8/1
  Constant23/1 -> GreaterThan2/2
  [VTQD_GearActualPosn_enum] -> Equal/1
  Constant29/1 -> Equal/2
  VTQD_GearActualPosn_enum/1 -> [VTQD_GearActualPosn_enum]
  Constant30/1 -> Equal1/2
  [VTQD_FrTMRotateDirction_enum] -> Equal1/1
  Equal/1 -> Logical Operator/1
  Equal1/1 -> Logical Operator/2
  Equal3/1 -> Logical Operator2/2
  Equal2/1 -> Logical Operator2/1
  [VTQD_FrTMRotateDirction_enum] -> Equal3/1
  Constant32/1 -> Equal3/2
  Constant31/1 -> Equal2/2
  [VTQD_GearActualPosn_enum] -> Equal2/1
  Logical Operator2/1 -> Logical Operator1/2
  Logical Operator/1 -> Logical Operator1/1
  Logical Operator1/1 -> LiuzgSwitch11/2
  Constant34/1 -> LiuzgSwitch11/1
  Constant33/1 -> LiuzgSwitch11/3
  LiuzgSwitch11/1 -> [FrDirectionIndicator]
  [VINP_FrTMSpd_rpm] -> Abs/1
  [VINP_RrTMSpd_rpm] -> Abs1/1
  Product2/1 -> Gain/1
  Product3/1 -> Gain2/1
  Gain2/1 -> [VTQD_RrShaftSpd_rpm], VTQD_RrShaftSpd_rpm/1  "VTQD_RrShaftSpd_rpm"
  Gain/1 -> [VTQD_FrShaftSpd_rpm], VTQD_FrShaftSpd_rpm/1  "VTQD_FrShaftSpd_rpm"
  LiuzgSwitch12/1 -> VTQD_TMRotateDirction_enum/1  "VTQD_TMRotateDirction_enum"
  [VTQD_RrTMRotateDirction_enum] -> LiuzgSwitch12/3
  [VTQD_FrTMRotateDirction_enum] -> LiuzgSwitch12/1
  Constant6/1 -> Equal4/2
  [VPMM_DrivetrainSelect_enum] -> Equal4/1
  Equal4/1 -> LiuzgSwitch12/2
  Abs/1 -> Product2/1
  Abs1/1 -> Product3/2
  LiuzgSwitch13/1 -> [RrDirectionIndicator]
  Constant38/1 -> LiuzgSwitch13/3
  Constant39/1 -> LiuzgSwitch13/1
  Logical Operator4/1 -> LiuzgSwitch13/2
  Logical Operator3/1 -> Logical Operator4/1
  Logical Operator5/1 -> Logical Operator4/2
  [VTQD_GearActualPosn_enum] -> Equal7/1
  Constant36/1 -> Equal7/2
  Constant37/1 -> Equal9/2
  [VTQD_RrTMRotateDirction_enum] -> Equal9/1
  Equal7/1 -> Logical Operator5/1
  Equal9/1 -> Logical Operator5/2
  Equal6/1 -> Logical Operator3/2
  Equal5/1 -> Logical Operator3/1
  [VTQD_RrTMRotateDirction_enum] -> Equal6/1
  Constant35/1 -> Equal6/2
  Constant10/1 -> Equal5/2
  [VTQD_GearActualPosn_enum] -> Equal5/1
  [FrDirectionIndicator] -> Product2/2
  [RrDirectionIndicator] -> Product3/1
  VDHP_LowIdleAccPedal_flg/1 -> LiuzgSwitch15/3
  Constant43/1 -> LiuzgSwitch15/1
  Constant42/1 -> LiuzgSwitch15/2
  LiuzgSwitch15/1 -> VTQD_LowIdleAccPedal_flg/1, [VTQD_LowIdleAccPedal_flg]  "VTQD_LowIdleAccPedal_flg"
  OR/1 -> [VTQD_BrkSwSta_flg], VTQD_BrkSwSta_flg/1  "VTQD_BrkSwSta_flg"
  VINP_BrakeSWGPIO_flg/1 -> OR/2
  LiuzgSwitch5/1 -> OR/1
  Constant52/1 -> Switch4/3
  Constant53/1 -> Equal10/2
  [VTQD_GearActualPosn_enum] -> Equal10/1
  Equal10/1 -> Switch4/2
  Constant51/1 -> Switch4/1
  [VTQD_GearActualPosn_enum] -> Equal11/1
  Constant54/1 -> Equal11/2
  Equal11/1 -> Switch5/2
  Switch4/1 -> Switch5/3
  Constant50/1 -> Switch5/1
  Switch5/1 -> Switch6/3
  Constant55/1 -> Switch6/1
  Equal12/1 -> Switch6/2
  Constant56/1 -> Equal12/2
  [VTQD_GearActualPosn_enum] -> Equal12/1
  [VTQD_GearActualPosn_enum] -> Equal13/1
  Constant58/1 -> Equal13/2
  Equal13/1 -> Switch9/2
  Constant57/1 -> Switch9/1
  Switch6/1 -> Switch9/3
  Switch9/1 -> VTQD_ShiftGearPosn_enum/1  "VTQD_ShiftGearPosn_enum"
  VPMM_DrivetrainSelect_enum/1 -> [VPMM_DrivetrainSelect_enum]
  Logical Operator6/1 -> LiuzgSwitch5/2
  VDHP_ActAPSPosn_pct/1 -> [VDHP_ActAPSPosn_pct]
  [VDHP_ActAPSPosn_pct] -> Less Than/1
  Constant40/1 -> Less Than/2
  Constant41/1 -> Less Than1/2
  Less Than/1 -> Logical Operator7/1
  Less Than1/1 -> Logical Operator7/2
  Constant62/1 -> LiuzgSwitch17/3
  [VPMM_DrivetrainSelect_enum] -> Equal23/1
  Equal23/1 -> AND9/2
  Constant59/1 -> Equal17/2
  Constant49/1 -> Equal19/2
  AND2/1 -> LiuzgSwitch16/2
  Equal19/1 -> AND2/2
  [VPMM_DrivetrainSelect_enum] -> Equal19/1
  [VPMM_DrivetrainSelect_enum] -> Equal18/1
  Constant48/1 -> Equal18/2
  Equal18/1 -> AND2/1
  Equal17/1 -> AND9/1
  Constant60/1 -> Equal23/2
  Constant61/1 -> LiuzgSwitch16/3
  [VPMM_DrivetrainSelect_enum] -> Equal17/1
  AND9/1 -> LiuzgSwitch17/2
  LiuzgSwitch19/1 -> VTQD_FrActvDmpDisabReq_flg/1  "VTQD_FrActvDmpDisabReq_flg"
  LiuzgSwitch20/1 -> VTQD_RrActvDmpDisabReq_flg/1  "VTQD_RrActvDmpDisabReq_flg"
  LiuzgSwitch16/1 -> LiuzgSwitch19/3
  LiuzgSwitch17/1 -> LiuzgSwitch20/3
  Constant64/1 -> LiuzgSwitch19/1
  Constant67/1 -> LiuzgSwitch19/2
  Constant63/1 -> LiuzgSwitch20/1
  Constant68/1 -> LiuzgSwitch20/2
  [VPMM_DrivetrainSelect_enum] -> Equal14/1
  Equal16/1 -> If/3
  AWDMCUReadyExt_flg/1(VTQD_AWDMCUReadyExt_flg) -> Merge/1
  Constant72/1 -> Equal16/2
  Merge/1 -> VTQD_MCUReady4Ext_flg/1  "VTQD_MCUReady4Ext_flg"
  Constant75/1 -> Equal14/2
  FWDMCUReadyExt_flg/1(VTQD_FWDMCUReadyExt_flg) -> Merge/2
  [VPMM_DrivetrainSelect_enum] -> Equal15/1
  Equal15/1 -> If/2
  If/3 -> RWDMCUReadyExt_flg/Action
  RWDMCUReadyExt_flg/1(VTQD_RWDMCUReadyExt_flg) -> Merge/3
  [VPMM_DrivetrainSelect_enum] -> Equal16/1
  If/1 -> AWDMCUReadyExt_flg/Action
  If/2 -> FWDMCUReadyExt_flg/Action
  Constant76/1 -> Equal15/2
  Equal14/1 -> If/1
  VINP_CreepSW_flg/1 -> Terminator/1
  VINP_IVIPWModeReq_enum/1 -> [VINP_IVIPWModeReq_enum]
  [VINP_IVIPWModeReq_enum] -> Equal21/1
  Equal21/1 -> LiuzgSwitch21/2
  LiuzgSwitch22/1 -> LiuzgSwitch21/3
  [VINP_IVIPWModeReq_enum] -> Equal22/1
  Equal22/1 -> LiuzgSwitch22/2
  Constant47/1 -> Equal21/2
  Constant70/1 -> Equal22/2
  Constant71/1 -> LiuzgSwitch21/1
  Constant69/1 -> LiuzgSwitch22/1
  LiuzgSwitch21/1 -> Switch3/3
  Constant46/1 -> LiuzgSwitch22/3
  [VDHP_ActAPSPosn_pct] -> Data Type Conversion2/1
  [VTQD_RDCActive_enum] -> Equal20/1
  Equal20/1 -> VTQD_RollRegenDisable_flg/1, [VTQD_RollRegenDisableReq_flg]  "VTQD_RollRegenDisable_flg"
  Constant2/1 -> Equal20/2
  VINP_FrEDURealTMTq_Nm/1 -> [VINP_FrEDURealTMTq_Nm]
  task_time_s/1 -> [task_time_s]
  VINP_MCUWarnR_enum/1 -> [VINP_MCUWarnR_enum]
  VINP_MCUWarnF_enum/1 -> [VINP_MCUWarnF_enum]
  VINP_RrEDURealTMTq_Nm/1 -> [VINP_RrEDURealTMTq_Nm]
  [VINP_MCUWarnR_enum] -> AWDMCUReadyExt_flg/2(VINP_RrMCUErr_enum)
  [VINP_MCUWarnF_enum] -> FWDMCUReadyExt_flg/1(VINP_FrMCUErr_enum)
  [VINP_MCUWarnF_enum] -> AWDMCUReadyExt_flg/1(VINP_FrMCUErr_enum)
  [VINP_MCUWarnR_enum] -> RWDMCUReadyExt_flg/1(VINP_RrMCUErr_enum)
  VINP_IVICreepSWReq_flg/1 -> [VINP_IVICreepSWReq_flg]
  VPMM_SysPowerMode_enum/1 -> [VPMM_SysPowerMode_enum]
  VTQD_OPDOn2Off_flg/1 -> [VTQD_OPDOn2Off_flg]
  VINP_RegenMode_enum/1 -> [VINP_RegenMode_enum]
  [VINP_IVICreepSWReq_flg] -> Detect Decrease4/1
  [VPMM_SysPowerMode_enum] -> Chart/1(VPMM_SysPowerMode_enum)
  [VTQD_OPDOn2Off_flg] -> Chart/4(VTQD_OPDOn2Off_flg)
  [VINP_RegenMode_enum] -> Chart/5(VINP_RegenMode_enum)
  [VTQD_LastCreepON_flg] -> Chart/6(VTQD_LastCreepON_flg)
  Detect Decrease4/1 -> Chart/7(VINP_IVICreepSWReq_flg)
  Constant80/1 -> Chart/3(KTQD_CreepSW_flg_ovrdval)
  Constant79/1 -> Chart/2(KTQD_CreepSW_flg_ovrdflg)
  Chart/1(VTQD_CreepON_flg) -> Unit Delay1/1, VTQD_CreepON_flg/1  "VTQD_CreepON_flg"
  Unit Delay1/1 -> [VTQD_LastCreepON_flg]
  VINP_FrntAxlTrqReqBrk_Nm/1 -> [VINP_FrntAxlTrqReqBrk_Nm]
  VINP_RearAxlTrqReqBrk_Nm/1 -> [VINP_RearAxlTrqReqBrk_Nm]
  VINP_FrRBCActive_flg/1 -> [VINP_FrRBCActive_flg]
  VINP_RrRBCActive_flg/1 -> [VINP_RrRBCActive_flg]
  VVMC_ADASActive_flg/1 -> [VVMC_ADASActive_flg]
  VINP_ACCRequiredAccel_mps2/1 -> [VINP_ACCRequiredAccel_mps2]
  VINP_VehSpeed_kph/1 -> [VINP_VehSpeed_kph]
  [VINP_VehSpeed_kph] -> Less Than1/1
  [VINP_FrntAxlTrqReqBrk_Nm] -> Equal24/1
  Constant9/1 -> Equal24/2
  Constant24/1 -> Equal25/2
  [VINP_FrEDURealTMTq_Nm] -> Equal25/1
  [VINP_FrRBCActive_flg] -> Logical Operator9/1
  [VINP_ACCRequiredAccel_mps2] -> Equal26/1
  Constant25/1 -> Equal26/2
  Equal24/1 -> Logical Operator10/1
  Equal25/1 -> Logical Operator10/2
  Logical Operator10/1 -> Logical Operator11/1
  Logical Operator9/1 -> Logical Operator11/2
  Equal26/1 -> Logical Operator11/3
  Logical Operator11/1 -> SR_Latch1/2
  [VVMC_ADASActive_flg] -> Logical Operator12/1
  [VINP_FrRBCActive_flg] -> Logical Operator12/2
  Logical Operator12/1 -> SR_Latch1/1
  SR_Latch1/1 -> Logical Operator17/2
  Logical Operator17/1 -> [VTQD_FrADASRegMCUDmDis_flg]  "VTQD_FrADASRegMCUDmDis_flg"
  [VINP_VehSpeed_kph] -> Relay/1
  Data Type Conversion/1 -> Logical Operator17/1  "VTQD_FrMCUDmDisSpd_flg"
  Data Type Conversion1/1 -> Logical Operator18/1  "VTQD_RrMCUDmDisSpd_flg"
  [VINP_VehSpeed_kph] -> Relay1/1
  Logical Operator18/1 -> [VTQD_RrADASRegMCUDmDis_flg]  "VTQD_RrADASRegMCUDmDis_flg"
  SR_Latch2/1 -> Logical Operator18/2
  Logical Operator15/1 -> SR_Latch2/1
  [VINP_RrRBCActive_flg] -> Logical Operator15/2
  [VVMC_ADASActive_flg] -> Logical Operator15/1
  Logical Operator14/1 -> SR_Latch2/2
  Equal29/1 -> Logical Operator14/3
  Logical Operator16/1 -> Logical Operator14/2
  Logical Operator13/1 -> Logical Operator14/1
  Equal28/1 -> Logical Operator13/2
  Equal27/1 -> Logical Operator13/1
  Constant44/1 -> Equal29/2
  [VINP_ACCRequiredAccel_mps2] -> Equal29/1
  [VINP_RrRBCActive_flg] -> Logical Operator16/1
  [VINP_RrEDURealTMTq_Nm] -> Equal28/1
  Constant27/1 -> Equal28/2
  Constant65/1 -> Equal27/2
  [VINP_RearAxlTrqReqBrk_Nm] -> Equal27/1
  [VTQD_FrADASRegMCUDmDis_flg] -> Logical Operator19/1
  Logical Operator7/1 -> [VTQD_MCUDmpDisabReq_flg]  "VTQD_MCUDmpDisabReq_flg"
  [VTQD_MCUDmpDisabReq_flg] -> Logical Operator19/2
  Logical Operator19/1 -> LiuzgSwitch16/1
  [VTQD_MCUDmpDisabReq_flg] -> Logical Operator8/2
  [VTQD_RrADASRegMCUDmDis_flg] -> Logical Operator8/1
  Logical Operator8/1 -> LiuzgSwitch17/1
  Relay/1 -> Data Type Conversion/1
  Relay1/1 -> Data Type Conversion1/1
  VVMC_ACCPedalOvrd_flg/1 -> [VVMC_ACCPedalOvrd_flg]
  VTQD_AfterAvailableTqDemFr_Nm/1 -> [VTQD_AfterAvailableTqDemFr_Nm]
  VTQD_AfterAvailableTqDemRr_Nm/1 -> [VTQD_AfterAvailableTqDemRr_Nm]
  VVMC_ADASWhlTqReq_Nm/1 -> [VVMC_ADASWhlTqReq_Nm]
  [VTQD_BrkSwSta_flg] -> VehWeightEst/10(VTQD_BrkSwSta_flg)
  [VINP_RCenterSeatBeltCmd_flg] -> VehWeightEst/21(VINP_RCenterSeatBeltCmd_flg)
  [VINP_RDriverSeatBeltCmd_flg] -> VehWeightEst/20(VINP_RDriverSeatBeltCmd_flg)
  [VVMC_EstSlope_Deg] -> VehWeightEst/13(VVMC_EstSlope_Deg)
  [VINP_FrRBCActive_flg] -> VehWeightEst/12(VINP_FrRBCActive_flg)
  [VTQD_GearActualPosn_enum] -> VehWeightEst/5(VTQD_GearActualPosn_enum)
  [VTQD_AfterAvailableTqDemRr_Nm] -> VehWeightEst/1(VTQD_AfterAvailableTqDemRr_Nm)
  VehWeightEst/1(VTQD_EstVehWeightResult_kg) -> VTQD_EstVehWeightResult_kg/1
  [VINP_RrRBCActive_flg] -> VehWeightEst/11(VINP_RrRBCActive_flg)
  [VTQD_LowIdleAccPedal_flg] -> VehWeightEst/9(VTQD_LowIdleAccPedal_flg)
  [VINP_RegenMode_enum] -> VehWeightEst/8(VINP_RegenMode_enum)
  [VTQR_NoABSFEDUWhlTqReq_Nm] -> VehWeightEst/3(VTQR_NoABSFEDUWhlTqReq_Nm)
  [VTQR_NoABSREDUWhlTqReq_Nm] -> VehWeightEst/2(VTQR_NoABSREDUWhlTqReq_Nm)
  [VVMC_LongAcc_Gps] -> VehWeightEst/15(VVMC_LongAcc_Gps)
  [VINP_PsngrSeatBeltCmd_flg] -> VehWeightEst/19(VINP_PsngrSeatBeltCmd_flg)
  [VINP_DriverSeatBeltCmd_flg] -> VehWeightEst/18(VINP_DriverSeatBeltCmd_flg)
  [task_time_s] -> VehWeightEst/14(task_time_s)
  [VINP_VehSpeed_kph] -> VehWeightEst/6(VINP_VehSpeed_kph)
  [VINP_RrEDURealTMTq_Nm] -> VehWeightEst/17(VINP_RrEDURealTMTq_Nm)
  [VINP_FrEDURealTMTq_Nm] -> VehWeightEst/16(VINP_FrEDURealTMTq_Nm)
  [VTQD_AfterAvailableTqDemFr_Nm] -> VehWeightEst/4(VTQD_AfterAvailableTqDemFr_Nm)
  [VINP_RPsngrSeatBeltCmd_flg] -> VehWeightEst/22(VINP_RPsngrSeatBeltCmd_flg)
  [VTQD_RollRegenDisableReq_flg] -> VehWeightEst/7(VTQD_RollRegenDisableReq_flg)
  VINP_DriverSeatBeltCmd_flg/1 -> [VINP_DriverSeatBeltCmd_flg]
  VINP_PsngrSeatBeltCmd_flg/1 -> [VINP_PsngrSeatBeltCmd_flg]
  VTQR_NoABSREDUWhlTqReq_Nm/1 -> [VTQR_NoABSREDUWhlTqReq_Nm]
  VINP_RPsngrSeatBeltCmd_flg/1 -> [VINP_RPsngrSeatBeltCmd_flg]
  VINP_RCenterSeatBeltCmd_flg/1 -> [VINP_RCenterSeatBeltCmd_flg]
  VTQR_NoABSFEDUWhlTqReq_Nm/1 -> [VTQR_NoABSFEDUWhlTqReq_Nm]
  VINP_RDriverSeatBeltCmd_flg/1 -> [VINP_RDriverSeatBeltCmd_flg]
  VVMC_LongAcc_Gps/1 -> [VVMC_LongAcc_Gps]
  NOT/1 -> OR1/2
  Equal32/1 -> OR1/1
  [VINP_DOASta_flg] -> NOT/1
  VINP_RollModeSWCmd_enum/1 -> [VINP_RollModeSWCmd_enum]
  OR1/1 -> Switch12/2
  VINP_EPBCarWashMode_flg/1 -> [VINP_EPBCarWashMode_flg]
  [VTQD_EPBCarWashMode_flg] -> Delay/1
  [VINP_EPBCarWashMode_flg] -> Switch12/3
  Delay/1 -> AND/2
  Switch12/1 -> [VTQD_EPBCarWashMode_flg]  "VTQD_EPBCarWashMode_flg"
  [VINP_RollModeSWCmd_enum] -> Detect Decrease5/1
  [VINP_SCPSystemMode_enum] -> Equal32/1
  SR_Latch3/1 -> Switch12/1
  VINP_SCPSystemMode_enum/1 -> [VINP_SCPSystemMode_enum]
  Constant66/1 -> Equal32/2
  Detect Decrease5/1 -> AND/1, SR_Latch3/1
  VINP_DOASta_flg/1 -> [VINP_DOASta_flg]
  AND/1 -> SR_Latch3/2
  [VTQD_EPBCarWashMode_flg] -> VTQD_EPBCarWashMode_flg/1
  Data Type Conversion2/1 -> VTQD_ActAPSPosn_pct/1  "VTQD_ActAPSPosn_pct"
  VVMC_EstSlope_Deg/1 -> [VVMC_EstSlope_Deg]
  Relational Operator/1 -> AND1/1
  Logical Operator22/1 -> Switch1/1
  [VINP_ACCRequiredAccel_mps2] -> Relational Operator5/1
  DelayEnable4/1 -> Switch7/2
  AND1/1 -> DelayEnable4/1
  [task_time_s] -> DelayEnable4/3
  Relational Operator5/1 -> AND1/2
  Switch/1 -> VTQD_EquivAccPedalSWSta_flg/1  "VTQD_EquivAccPedalSWSta_flg"
  Constant45/1 -> Switch7/3
  Constant26/1 -> Switch7/1
  Constant8/1 -> Relational Operator/2
  [VVMC_ADASWhlTqReq_Nm] -> Relational Operator/1
  Switch7/1 -> Switch1/3
  [VTQD_LowIdleAccPedal_flg] -> Logical Operator21/1
  Switch1/1 -> Switch/1
  [VVMC_ADASActive_flg] -> Switch/2
  Logical Operator21/1 -> Switch/3
  [VVMC_ACCPedalOvrd_flg] -> Switch1/2
  Constant93/1 -> DelayEnable4/2
  [VTQD_LowIdleAccPedal_flg] -> Logical Operator22/1
  Constant97/1 -> Switch14/1
  [VTQD_IVIPwrLock_flg] -> Switch14/2
  Delay8/1 -> AND5/2
  Switch14/1 -> VTQD_IVIPwrLockSta_enum/1  "VTQD_IVIPwrLockSta_enum"
  Constant98/1 -> Switch14/3
  [VTQD_IVIPwrLock_flg] -> Delay8/1
  AND4/1 -> [VTQD_IVIPwrLock_flg], VTQD_IVIPwrLock_flg/1  "VTQD_IVIPwrLock_flg"
  [VINP_IVIPwrLockSW_enum] -> Equal34/1
  Equal34/1 -> Detect Decrease/1
  AND5/1 -> SR_Latch6/2
  Detect Decrease/1 -> AND5/1, SR_Latch6/1
  Constant96/1 -> Equal34/2
  VINP_IVIPwrLockSW_enum/1 -> [VINP_IVIPwrLockSW_enum]
  Constant85/1 -> Relational Operator5/2
  [VVMC_RWDRDCActive_enum] -> Data Type Conversion3/1
  Data Type Conversion3/1 -> VTQD_RDCActive_enum/1, [VTQD_RDCActive_enum]  "VTQD_RDCActive_enum"
  VVMC_RWDRDCActive_enum/1 -> [VVMC_RWDRDCActive_enum]
  AND3/1 -> Switch8/2
  Delay3/1 -> SR_Latch/2
  [VTQD_RegenModeChange_flg] -> AND3/2
  Abs2/1 -> Relational Operator1/1
  [VTQD_LowIdleAccPedal_flg] -> Switch11/3
  Switch11/1 -> [VTQD_RngChgReset_flg]  "VTQD_RngChgReset_flg"
  [VTQD_RegenMode_enum] -> VTQD_RegenMode_enum/1
  Constant73/1 -> Relational Operator1/2
  Constant74/1 -> AND3/1
  [VTQD_RngChgReset_flg] -> Delay3/1
  [VTQD_RgnModeChgAPSPosn_pct] -> Add/2
  [VDHP_ActAPSPosn_pct] -> Add/1
  Switch8/1 -> [VTQD_RegenMode_enum], Delay1/1  "VTQD_RegenMode_enum"
  Add/1 -> Abs2/1
  Switch10/1 -> [VTQD_RgnModeChgAPSPosn_pct], Delay2/1  "VTQD_RgnModeChgAPSPosn_pct"
  Constant1/1 -> Switch11/2
  Delay2/1 -> Switch10/1
  Relational Operator1/1 -> Switch11/1
  Delay1/1 -> Switch8/1
  [VTQD_RegenModeChange_flg] -> Switch10/2
  [VINP_RegenMode_enum] -> Switch8/3
  SR_Latch/1 -> [VTQD_RegenModeChange_flg]  "VTQD_RegenModeChange_flg"
  [VINP_RegenMode_enum] -> Detect Change/1
  [VDHP_ActAPSPosn_pct] -> Switch10/3
  Detect Change/1 -> SR_Latch/1
  Delay4/1 -> AND4/2
  SR_Latch6/1 -> AND4/1
  Constant77/1 -> Equal30/2
  [VTQD_GearActualPosn_enum] -> Equal30/1
  Equal30/1 -> Delay4/1
